simulink model "Main_JA"  (R2021b)
settings: Solver=VariableStepAuto  StartTime=0.0  StopTime=5  RelTol=1e-3
undefined symbols (not defined in the file): CM_FUEL_b, cmFuel_cmL, g, m_dot, m_iFuel, W_lander, W_LANDER
libraries: shared6dof x2, matrix_library x2
settings Model: Creator=josepfamador  LastModifiedBy=josepfamador
settings DebuggingCC: SignalRangeChecking=warning

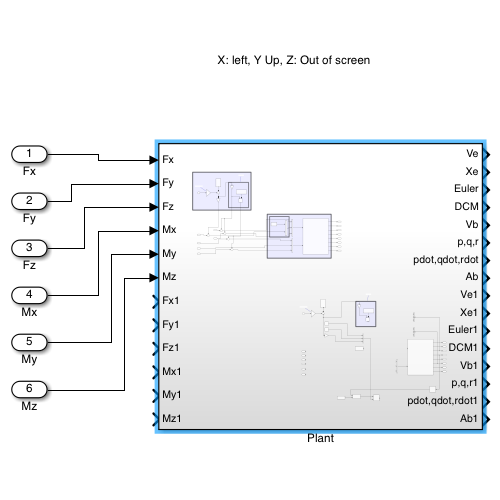
[thumbnail: Simulink's stored preview of the top-level diagram]
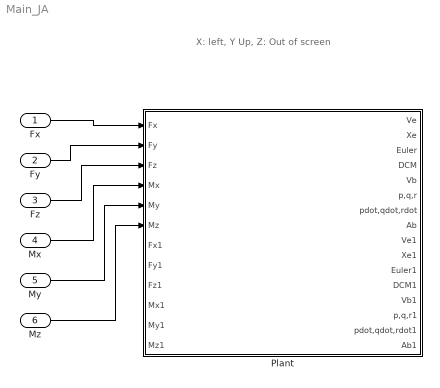
== system Main_JA ==
  note: X: left, Y Up, Z: Out of screen
  Fx : Inport
  Fy : Inport  Port=2
  Fz : Inport  Port=3
  Mx : Inport  Port=4
  My : Inport  Port=5
  Mz : Inport  Port=6
  Plant : Subsystem
  wires:
  Fx/1 -> Plant/1(Fx)
  Fy/1 -> Plant/2(Fy)
  Fz/1 -> Plant/3(Fz)
  Mx/1 -> Plant/4(Mx)
  My/1 -> Plant/5(My)
  Mz/1 -> Plant/6(Mz)

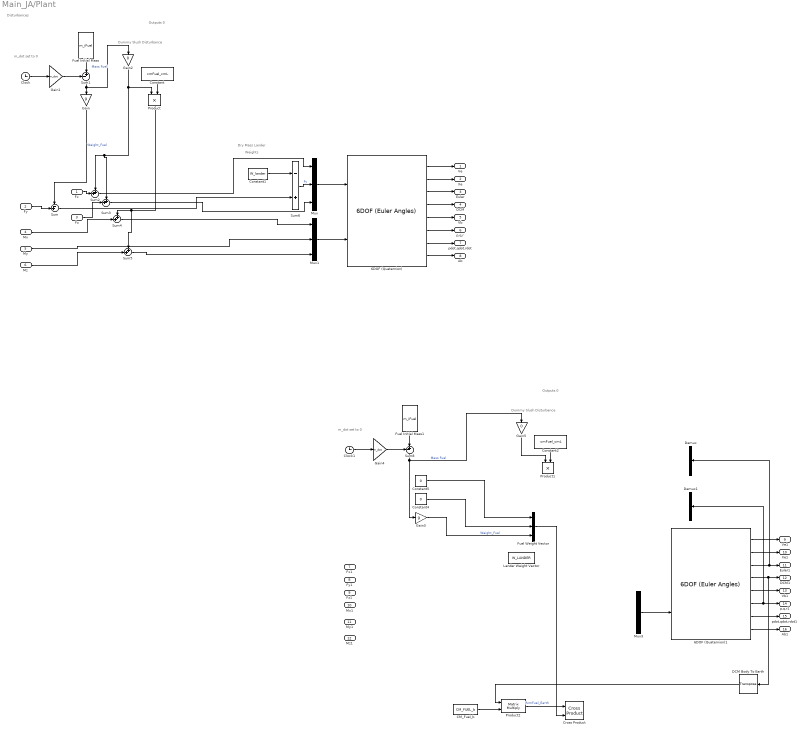
== system Main_JA/Plant ==
  note: Weights
  note: Dummy Slush Disturbance
  note: Disturbances
  note: Dry Mass Lander
  note: Outputs 0
  note: m_dot set to 0
  note: Outputs 0
  note: m_dot set to 0
  note: Dummy Slush Disturbance
  Fx : Inport
  Fy : Inport  Port=2
  Fz : Inport  Port=3
  Mx : Inport  Port=4
  My : Inport  Port=5
  Mz : Inport  Port=6
  Fx1 : Inport  Port=7
  Fy1 : Inport  Port=8
  Fz1 : Inport  Port=9
  Mx1 : Inport  Port=10
  My1 : Inport  Port=11
  Mz1 : Inport  Port=12
  6DOF (Quaternion) : shared6dof/6DOF (Euler Angles)  units=Metric (MKS)  mtype=Fixed  rep=Quaternion  xme_0=[0 0 0]  Vm_0=[0 0 0]  eul_0=[0 0 0]  pm_0=[0 0 0]  mass_0=1.0  mass_e=0.5  mass_f=2.0  inertia=eye(3)  inertia_e=eye(3)  inertia_f=2*eye(3)  k_quat=1.0  vre_flag=on  abi_flag=off  aMode=0  xme_statename='Position_earth'  Vm_statename=''  eul_statename=''  quat_statename=''  pm_statename=''  mass_statename=''
      settings: SourceProductBaseCode=AE,PW,DR,MT,UV,VE
  6DOF (Quaternion)1 : shared6dof/6DOF (Euler Angles)  units=Metric (MKS)  mtype=Fixed  rep=Euler Angles  xme_0=[0 0 0]  Vm_0=[0 0 0]  eul_0=[0 0 0]  pm_0=[0 0 0]  mass_0=1.0  mass_e=0.5  mass_f=2.0  inertia=eye(3)  inertia_e=eye(3)  inertia_f=2*eye(3)  k_quat=1.0  vre_flag=on  abi_flag=off  aMode=0  xme_statename='Position_earth'  Vm_statename=''  eul_statename=''  quat_statename=''  pm_statename=''  mass_statename=''
      settings: SourceProductBaseCode=AE,PW,DR,MT,UV,VE
  CM_Fuel_b : Constant  Value=CM_FUEL_b
  Clock : Clock
  Clock1 : Clock
  Constant : Constant  Value=cmFuel_cmL
  Constant1 : Constant  Value=W_lander
  Constant2 : Constant  Value=cmFuel_cmL
  Constant4 : Constant  Value=0
  Constant5 : Constant  Value=0
  Cross Product : matrix_library/Cross Product
      settings: SourceProductBaseCode=SL
  DCM Body To Earth : matrix_library/Transpose
      settings: SourceProductBaseCode=SL
  Demux : Demux  Outputs=3
  Demux1 : Demux  Outputs=3
  Fuel Initial Mass : Constant  Value=m_iFuel
  Fuel Initial Mass1 : Constant  Value=m_iFuel
  Fuel Weight Vector : Mux  Inputs=3
  Gain : Gain  Gain=g
  Gain1 : Gain  Gain=m_dot
  Gain2 : Gain  Gain=0
  Gain3 : Gain  Gain=g
  Gain4 : Gain  Gain=m_dot
  Gain5 : Gain  Gain=0
  Lander Weight Vector : Constant  Value=W_LANDER
  Mux : Mux  Inputs=3
  Mux1 : Mux  Inputs=3
  Mux3 : Mux  Inputs=3
  Product : Product
  Product1 : Product
  Product2 : Product  Multiplication=Matrix(*)
  Sum : Sum  Inputs=-+|
  Sum1 : Sum  Inputs=-+|
  Sum{2..5} (4 alike) : Sum  Inputs=++|
  Sum6 : Sum  Inputs=-+
  Sum8 : Sum  Inputs=-+|
  Ve : Outport
  Xe : Outport  Port=2
  Euler : Outport  Port=3
  DCM : Outport  Port=4
  Vb : Outport  Port=5
  p,q,r : Outport  Port=6
  pdot,qdot,rdot : Outport  Port=7
  Ab : Outport  Port=8
  Ve1 : Outport  Port=9
  Xe1 : Outport  Port=10
  Euler1 : Outport  Port=11
  DCM1 : Outport  Port=12
  Vb1 : Outport  Port=13
  p,q,r1 : Outport  Port=14
  pdot,qdot,rdot1 : Outport  Port=15
  Ab1 : Outport  Port=16
  wires:
  6DOF (Quaternion)/4 -> DCM/1
  6DOF (Quaternion)/2 -> Xe/1
  6DOF (Quaternion)/5 -> Vb/1
  Product/1 -> Sum4/1, Sum5/1
  6DOF (Quaternion)/6 -> p,q,r/1
  6DOF (Quaternion)/1 -> Ve/1
  Gain2/1 -> Sum2/1, Sum3/1, Product/1
  Fy/1 -> Sum/2
  Fx/1 -> Sum2/2
  6DOF (Quaternion)/3 -> Euler/1
  Fz/1 -> Sum3/2
  6DOF (Quaternion)/7 -> pdot,qdot,rdot/1
  6DOF (Quaternion)/8 -> Ab/1
  Mx/1 -> Sum4/2
  Mz/1 -> Sum5/2
  My/1 -> Mux1/2
  Sum5/1 -> Mux1/3
  Sum2/1 -> Mux/1
  Sum3/1 -> Mux/3
  Mux1/1 -> 6DOF (Quaternion)/2
  Sum4/1 -> Mux1/1
  Mux/1 -> 6DOF (Quaternion)/1
  Fuel Initial Mass/1 -> Sum1/2
  Sum1/1 -> Gain2/1, Gain/1  "Mass Fuel"
  Gain/1 -> Sum/1  "Weight_Fuel"
  Gain1/1 -> Sum1/1
  Clock/1 -> Gain1/1
  Constant/1 -> Product/2
  Constant1/1 -> Sum6/1
  Sum/1 -> Sum6/2
  Sum6/1 -> Mux/2  "Fy"
  6DOF (Quaternion)1/1 -> Ve1/1
  Gain5/1 -> Product1/1
  6DOF (Quaternion)1/3 -> Demux/1, Euler1/1
  6DOF (Quaternion)1/8 -> Ab1/1
  Fuel Initial Mass1/1 -> Sum8/2
  Mux3/1 -> 6DOF (Quaternion)1/2
  Sum8/1 -> Gain5/1, Gain3/1  "Mass Fuel"
  Clock1/1 -> Gain4/1
  Gain4/1 -> Sum8/1
  6DOF (Quaternion)1/6 -> Demux1/1, p,q,r1/1
  Constant2/1 -> Product1/2
  6DOF (Quaternion)1/4 -> DCM1/1, DCM Body To Earth/1
  6DOF (Quaternion)1/2 -> Xe1/1
  6DOF (Quaternion)1/5 -> Vb1/1
  6DOF (Quaternion)1/7 -> pdot,qdot,rdot1/1
  Gain3/1 -> Fuel Weight Vector/3  "Weight_Fuel"
  Constant4/1 -> Fuel Weight Vector/2
  Constant5/1 -> Fuel Weight Vector/1
  CM_Fuel_b/1 -> Product2/2
  DCM Body To Earth/1 -> Product2/1
  Product2/1 -> Cross Product/1  "RcmFuel_Earth"
  Fuel Weight Vector/1 -> Cross Product/2
